simulink model "model_r2016b"  (R2016b)
settings: Solver=VariableStepAuto  StartTime=0.0  StopTime=10.0  RelTol=1e-6
values from neighbouring files (symbols this model uses):
  a = 1.1    [Youla_controller.mat]    (also in parameters.m)
  b = 1.68    [Youla_controller.mat]    (also in parameters.m)
  b_hsf = 22.9183118052    [Youla_controller.mat]    (also in extendedKalmanFilter.m = obj.b_hsf; parameters.m; unscentedKalmanFilter.m = obj.b_hsf)
  b_hsf_RL = 45.8366236105    [Youla_controller.mat]    (also in parameters.m)
  b_hsf_RR = 45.8366236105    [Youla_controller.mat]    (also in parameters.m)
  b_sf_R = 45.8366236105    [Youla_controller.mat]    (also in parameters.m)
  chassis_state_init = [U_0 0 0 U_0/rw U_0/rw U_0/rw U_0/rw 0 0 0]    [main.m]
  Cx = 43302.5    [Youla_controller.mat]    (also in parameters.m; sandbox.m = CRx)
  Cy = 28427.8739632    [Youla_controller.mat]    (also in parameters.m; sandbox.m = CRy)
  DFFy = 310.189835229    [Youla_controller.mat]    (also in parameters.m)
  DFRy = 203.100487352    [Youla_controller.mat]    (also in parameters.m)
  DFx = 143.09352518    [Youla_controller.mat]    (also in parameters.m)
  fFLz0 = 4535.18417266    [Youla_controller.mat]    (also in parameters.m)
  fFRz0 = 4535.18417266    [Youla_controller.mat]    (also in parameters.m)
  fRLz0 = 2969.46582734    [Youla_controller.mat]    (also in extendedKalmanFilter.m = obj.fRLz0; parameters.m; unscentedKalmanFilter.m = obj.fRLz0)
  fRRz0 = 2969.46582734    [Youla_controller.mat]    (also in extendedKalmanFilter.m = obj.fRRz0; parameters.m; unscentedKalmanFilter.m = obj.fRRz0)
  G = minreal(C*inv(s*eye(4)-A)*B + D,1e-9)    [Youla_design.m]    (also in extendedKalmanFilter.m = obj.G; parameters.m = 9.96488294314; unscentedKalmanFilter.m = obj.G)
  J_hsf = 0.009    [Youla_controller.mat]    (also in parameters.m)
  Jm_R = 0.0351    [Youla_controller.mat]    (also in extendedKalmanFilter.m = obj.Jm_R; parameters.m; unscentedKalmanFilter.m = obj.Jm_R)
  Jw = 0.9    [Youla_controller.mat]    (also in extendedKalmanFilter.m = obj.Jw; parameters.m; unscentedKalmanFilter.m = obj.Jw)
  Jy = 2315.3    [Youla_controller.mat]    (also in parameters.m)
  K_hsf = 2291.83118052    [Youla_controller.mat]    (also in extendedKalmanFilter.m = obj.K_hsf; parameters.m; unscentedKalmanFilter.m = obj.K_hsf)
  K_hsf_RL = 4583.66236105    [Youla_controller.mat]    (also in parameters.m)
  K_hsf_RR = 4583.66236105    [Youla_controller.mat]    (also in parameters.m)
  K_sf_R = 11459.1559026    [Youla_controller.mat]    (also in parameters.m)
  m = 1530    [Youla_controller.mat]    (also in extendedKalmanFilter.m = obj.m; parameters.m; unscentedKalmanFilter.m = obj.m)
  rear_axle_state_init = [G*U_0/rw 0]    [main.m]
  rw = 0.325    [Youla_controller.mat]    (also in extendedKalmanFilter.m = obj.rw; parameters.m; unscentedKalmanFilter.m = obj.rw)
  T = 1.55    [Youla_controller.mat]    (also in parameters.m; sandbox.m = 1.42857142857)
  U_0 = 100/3.6    (= 27.7777777778)    [main.m]
libraries: cstblocks x1
settings Model: Creator=louis  LastModifiedBy=louis

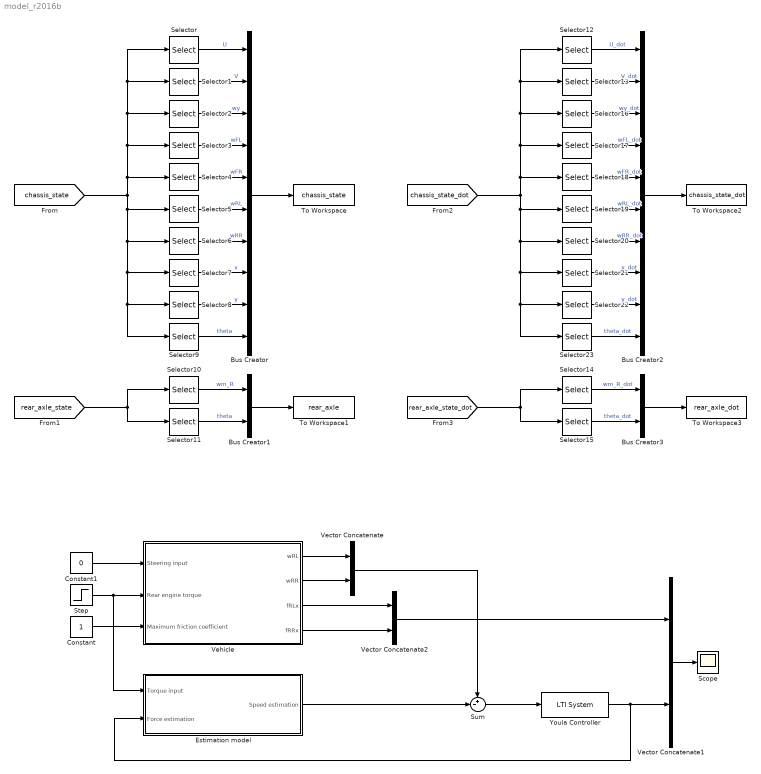
== system model_r2016b ==
  Bus Creator : BusCreator  Inputs=10
  Bus Creator1 : BusCreator  Inputs=2
  Bus Creator2 : BusCreator  Inputs=10
  Bus Creator3 : BusCreator  Inputs=2
  Constant : Constant
  Constant1 : Constant  Value=0
  Estimation model : Subsystem
  Scope : Scope
  Selector{,10,12,14} (4 alike) : Selector  IndexOptions=Index vector (dialog)  Indices=1  OutputSizes=1
  Selector{1,11,13,15} (4 alike) : Selector  IndexOptions=Index vector (dialog)  Indices=2  OutputSizes=1
  Selector16 : Selector  IndexOptions=Index vector (dialog)  Indices=3  OutputSizes=1
  Selector17 : Selector  IndexOptions=Index vector (dialog)  Indices=4  OutputSizes=1
  Selector18 : Selector  IndexOptions=Index vector (dialog)  Indices=5  OutputSizes=1
  Selector19 : Selector  IndexOptions=Index vector (dialog)  Indices=6  OutputSizes=1
  Selector2 : Selector  IndexOptions=Index vector (dialog)  Indices=3  OutputSizes=1
  Selector20 : Selector  IndexOptions=Index vector (dialog)  Indices=7  OutputSizes=1
  Selector21 : Selector  IndexOptions=Index vector (dialog)  Indices=8  OutputSizes=1
  Selector22 : Selector  IndexOptions=Index vector (dialog)  Indices=9  OutputSizes=1
  Selector23 : Selector  IndexOptions=Index vector (dialog)  Indices=10  OutputSizes=1
  Selector3 : Selector  IndexOptions=Index vector (dialog)  Indices=4  OutputSizes=1
  Selector4 : Selector  IndexOptions=Index vector (dialog)  Indices=5  OutputSizes=1
  Selector5 : Selector  IndexOptions=Index vector (dialog)  Indices=6  OutputSizes=1
  Selector6 : Selector  IndexOptions=Index vector (dialog)  Indices=7  OutputSizes=1
  Selector7 : Selector  IndexOptions=Index vector (dialog)  Indices=8  OutputSizes=1
  Selector8 : Selector  IndexOptions=Index vector (dialog)  Indices=9  OutputSizes=1
  Selector9 : Selector  IndexOptions=Index vector (dialog)  Indices=10  OutputSizes=1
  Step : Step  After=50  SampleTime=0
  Sum : Sum  Inputs=+-|
  To Workspace : ToWorkspace  VariableName=chassis_state  SaveFormat=Timeseries  SampleTime=-1
  To Workspace1 : ToWorkspace  VariableName=rear_axle  SaveFormat=Timeseries  SampleTime=-1
  To Workspace2 : ToWorkspace  VariableName=chassis_state_dot  SaveFormat=Timeseries  SampleTime=-1
  To Workspace3 : ToWorkspace  VariableName=rear_axle_dot  SaveFormat=Timeseries  SampleTime=-1
  Vector Concatenate : Concatenate
  Vector Concatenate1 : Concatenate
  Vector Concatenate2 : Concatenate
  Vehicle : Subsystem
  Youla Controller : cstblocks/LTI System  sys=Gc  IC=[]
  wires:
  [chassis_state] -> Selector4/1, Selector3/1, Selector2/1, Selector1/1, Selector/1, Selector5/1, Selector6/1, Selector7/1, Selector8/1, Selector9/1
  Selector/1 -> Bus Creator/1  "U"
  Selector9/1 -> Bus Creator/10  "theta"
  Selector8/1 -> Bus Creator/9  "y"
  Selector7/1 -> Bus Creator/8  "x"
  Selector6/1 -> Bus Creator/7  "wRR"
  Selector5/1 -> Bus Creator/6  "wRL"
  Bus Creator/1 -> To Workspace/1
  Selector1/1 -> Bus Creator/2  "V"
  Selector2/1 -> Bus Creator/3  "wy"
  Selector3/1 -> Bus Creator/4  "wFL"
  Selector4/1 -> Bus Creator/5  "wFR"
  Selector11/1 -> Bus Creator1/2  "theta"
  Bus Creator1/1 -> To Workspace1/1
  [rear_axle_state] -> Selector11/1, Selector10/1
  Selector10/1 -> Bus Creator1/1  "wm_R"
  Selector12/1 -> Bus Creator2/1  "U_dot"
  [chassis_state_dot] -> Selector18/1, Selector17/1, Selector16/1, Selector13/1, Selector12/1, Selector19/1, Selector20/1, Selector21/1, Selector22/1, Selector23/1
  Selector22/1 -> Bus Creator2/9  "y_dot"
  Selector20/1 -> Bus Creator2/7  "wRR_dot"
  Selector18/1 -> Bus Creator2/5  "wFR_dot"
  Bus Creator2/1 -> To Workspace2/1
  Selector16/1 -> Bus Creator2/3  "wy_dot"
  Bus Creator3/1 -> To Workspace3/1
  Selector13/1 -> Bus Creator2/2  "V_dot"
  Selector21/1 -> Bus Creator2/8  "x_dot"
  Selector23/1 -> Bus Creator2/10  "theta_dot"
  Selector19/1 -> Bus Creator2/6  "wRL_dot"
  [rear_axle_state_dot] -> Selector15/1, Selector14/1
  Selector15/1 -> Bus Creator3/2  "theta_dot"
  Selector17/1 -> Bus Creator2/4  "wFL_dot"
  Selector14/1 -> Bus Creator3/1  "wm_R_dot"
  Constant/1 -> Vehicle/3(Maximum friction coefficient)
  Constant1/1 -> Vehicle/1(Steering input)
  Step/1 -> Estimation model/1(Torque input), Vehicle/2(Rear engine torque)
  Vehicle/1(wRL) -> Vector Concatenate/1
  Vehicle/2(wRR) -> Vector Concatenate/2
  Sum/1 -> Youla Controller/1
  Vector Concatenate/1 -> Sum/1
  Youla Controller/1 -> Estimation model/2(Force estimation), Vector Concatenate1/2
  Estimation model/1(Speed estimation) -> Sum/2
  Vector Concatenate1/1 -> Scope/1
  Vehicle/3(fRLx) -> Vector Concatenate2/1
  Vehicle/4(fRRx) -> Vector Concatenate2/2
  Vector Concatenate2/1 -> Vector Concatenate1/1

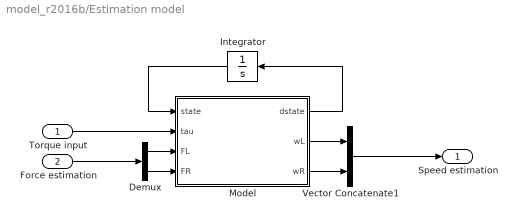
== system model_r2016b/Estimation model ==
  Torque input : Inport
  Force estimation : Inport  Port=2
  Demux : Demux  Outputs=2
  Integrator : Integrator  InitialCondition=[U_0/rw*G 0 U_0/rw U_0/rw]
  Model : MATLAB Function  TreatAsAtomicUnit=on
  Vector Concatenate1 : Concatenate
  Speed estimation : Outport
  wires:
  Demux/1 -> Model/3(FL)
  Vector Concatenate1/1 -> Speed estimation/1
  Integrator/1 -> Model/1(state)
  Model/3(wR) -> Vector Concatenate1/2
  Force estimation/1 -> Demux/1
  Model/2(wL) -> Vector Concatenate1/1
  Demux/2 -> Model/4(FR)
  Torque input/1 -> Model/2(tau)
  Model/1(dstate) -> Integrator/1

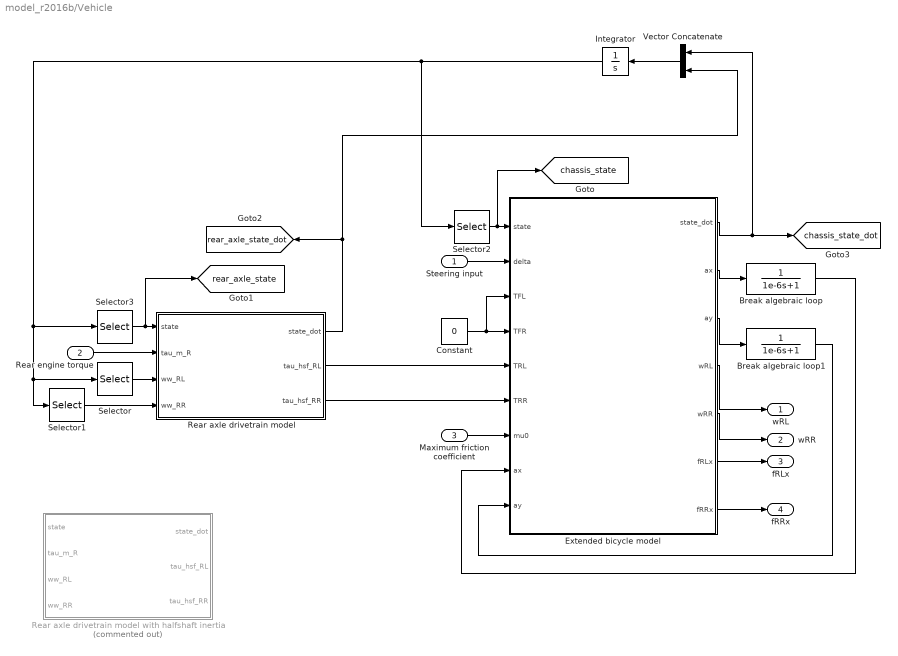
== system model_r2016b/Vehicle ==
  Steering input : Inport
  Rear engine torque : Inport  Port=2
  Maximum friction coefficient : Inport  Port=3
  Break algebraic loop : TransferFcn  Denominator=[1e-6 1]
  Break algebraic loop1 : TransferFcn  Denominator=[1e-6 1]
  Constant : Constant  Value=0
  Extended bicycle model : MATLAB Function  TreatAsAtomicUnit=on
  Integrator : Integrator  InitialCondition=[chassis_state_init rear_axle_state_init]
  Rear axle drivetrain model : MATLAB Function  TreatAsAtomicUnit=on
  Rear axle drivetrain model with halfshaft inertia : MATLAB Function  Commented=on  TreatAsAtomicUnit=on
  Selector : Selector  IndexOptions=Index vector (dialog)  Indices=[6]  OutputSizes=1
  Selector1 : Selector  IndexOptions=Index vector (dialog)  Indices=[7]  OutputSizes=1
  Selector2 : Selector  IndexOptions=Index vector (dialog)  Indices=[1:10]  OutputSizes=1
  Selector3 : Selector  IndexOptions=Index vector (dialog)  Indices=[11:12]  OutputSizes=1
  Vector Concatenate : Concatenate
  wRL : Outport
  wRR : Outport  Port=2
  fRLx : Outport  Port=3
  fRRx : Outport  Port=4
  tag scope: chassis_state=global, chassis_state_dot=global, rear_axle_state=global, rear_axle_state_dot=global
  wires:
  Maximum friction coefficient/1 -> Extended bicycle model/7(mu0)
  Steering input/1 -> Extended bicycle model/2(delta)
  Rear engine torque/1 -> Rear axle drivetrain model/2(tau_m_R)
  Extended bicycle model/3(ay) -> Break algebraic loop1/1
  Integrator/1 -> Selector2/1, Selector3/1, Selector1/1, Selector/1
  Rear axle drivetrain model/2(tau_hsf_RL) -> Extended bicycle model/5(TRL)
  Extended bicycle model/1(state_dot) -> Vector Concatenate/1, [chassis_state_dot]
  Rear axle drivetrain model/3(tau_hsf_RR) -> Extended bicycle model/6(TRR)
  Break algebraic loop1/1 -> Extended bicycle model/9("ay ")
  Break algebraic loop/1 -> Extended bicycle model/8("ax ")
  Extended bicycle model/2(ax) -> Break algebraic loop/1
  Constant/1 -> Extended bicycle model/4(TFR), Extended bicycle model/3(TFL)
  Selector1/1 -> Rear axle drivetrain model/4(ww_RR)
  Selector/1 -> Rear axle drivetrain model/3(ww_RL)
  Rear axle drivetrain model/1(state_dot) -> [rear_axle_state_dot], Vector Concatenate/2
  Vector Concatenate/1 -> Integrator/1
  Selector2/1 -> [chassis_state], Extended bicycle model/1(state)
  Selector3/1 -> [rear_axle_state], Rear axle drivetrain model/1(state)
  Extended bicycle model/4(wRL) -> wRL/1
  Extended bicycle model/5(wRR) -> wRR/1
  Extended bicycle model/6(fRLx) -> fRLx/1
  Extended bicycle model/7(fRRx) -> fRRx/1

== matlab function model_r2016b/Vehicle/Rear axle drivetrain model with halfshaft inertia ==
  data: state input; state_dot output; tau_m_R input; ww_RL input; ww_RR input; tau_hsf_RL output; tau_hsf_RR output; Jm_R parameter; J_hsf parameter; K_sf_R parameter; b_sf_R parameter; K_hsf_RL parameter; b_hsf_RL parameter; K_hsf_RR parameter; b_hsf_RR parameter; G parameter
function [state_dot, tau_hsf_RL, tau_hsf_RR] = ... 
    rearAxleModel(state, tau_m_R, ww_RL, ww_RR,...
    Jm_R, J_hsf, K_sf_R, b_sf_R, ...
    K_hsf_RL, b_hsf_RL, K_hsf_RR, b_hsf_RR, G) ...

%% Rename the states
wm_R         = state(1);    % Angular velocity of the rear shaft 
wh_RL        = state(2);    % Rear left halfshaft angular velocity
wh_RR        = state(3);    % Rear right halfshaft angular velocity
theta_hsf_RL = state(4);    % Rear left  axle halfshaft displacement 
theta_hsf_RR = state(5);    % Rear right axle halfshaft displacement
theta_sf_R   = state(6);    % Rear motor axle halfshaft displacement 

%% Shaft torque
tau_hsf_RL = K_hsf_RL * theta_hsf_RL + b_hsf_RL * (wh_RL - ww_RL); 
tau_hsf_RR = K_hsf_RR * theta_hsf_RR + b_hsf_RR * (wh_RR - ww_RR);
tau_sf_R   = K_sf_R   * theta_sf_R   + b_sf_R   * (wm_R - G/2*(wh_RL + wh_RR));

%% Compute the time derivatives
wm_rear_dot = 1/Jm_R * (tau_m_R - tau_sf_R);  
wh_RL_dot   = 1/J_hsf * (G*tau_sf_R/2 - tau_hsf_RL);
wh_RR_dot   = 1/J_hsf * (G*tau_sf_R/2 - tau_hsf_RR);
theta_hsf_RL_dot = wh_RL - ww_RL;
theta_hsf_RR_dot = wh_RR - ww_RR;
theta_sf_R_dot   = wm_R - G/2 * (wh_RL + wh_RR);

%% Return the state time derivative 
state_dot = [wm_rear_dot; wh_RL_dot; wh_RR_dot; theta_hsf_RL_dot;
    theta_hsf_RR_dot; theta_sf_R_dot];

end

== matlab function model_r2016b/Vehicle/Extended bicycle model ==
  data: state input; delta input; TFL input; TFR input; TRL input; TRR input; mu0 input; state_dot output; ax input; ay input; ax output; ay output; m parameter; Jy parameter; Jw parameter; a parameter; b parameter; T parameter; rw parameter; Cx parameter; Cy parameter; eps parameter; fFLz0 parameter; fFRz0 parameter; fRLz0 parameter; fRRz0 parameter; DFx parameter; DFFy parameter; DFRy parameter; wRL output; wRR output; fRLx output; fRRx output
function [state_dot,ax,ay,wRL,wRR,fRLx,fRRx] = vehicleEOM(state,delta,TFL,TFR,TRL,TRR,mu0,ax,ay,m,Jy,...
    Jw,a,b,T,rw,Cx,Cy,eps,fFLz0,fFRz0,fRLz0,fRRz0,DFx,DFFy,DFRy)

%% Rename the states
U     = state(1);
V     = state(2);
wy    = state(3);
wFL   = state(4);
wFR   = state(5);
wRL   = state(6);
wRR   = state(7);
theta = state(10);

%% Compute tire forces
% Wheel velocities
vFLxc = U - T*wy/2;
vFLyc = V + a*wy;
vFRxc = U + T*wy/2;
vFRyc = V + a*wy;
% Rotate to obtain velocities in the tire frame
vFLx =  vFLxc * cos(delta) + vFLyc * sin(delta);
vFLy = -vFLxc * sin(delta) + vFLyc * cos(delta);
vFRx =  vFRxc * cos(delta) + vFRyc * sin(delta);
vFRy = -vFRxc * sin(delta) + vFRyc * cos(delta);

vRLx = U - T*wy/2;
vRLy = V - b*wy;
vRRx = U + T*wy/2;
vRRy = V - b*wy;

% Wheel slip
% FL wheel
if abs(rw*wFL) > abs(vFLx)
    den = rw*wFL;
else
    den = vFLx;
end
if den == 0
    sFLx = 0;
else
    sFLx = -(vFLx - rw * wFL) / den;
end
% FR wheel
if abs(rw*wFR) > abs(vFRx)
    den = rw*wFR;
else
    den = vFRx;
end
if den == 0
    sFRx = 0;
else
    sFRx = -(vFRx - rw * wFR) / den;
end

% RL wheel
if abs(rw*wRL) > abs(vRLx)
    den = rw*wRL;
else
    den = vRLx;
end
if den == 0
    sRLx = 0;
else
    sRLx = -(vRLx - rw * wRL) / den;
end

% RR wheel
if abs(rw*wRR) > abs(vRRx)
    den = rw*wRR;
else
    den = vRRx;
end
if den == 0
    sRRx = 0;
else
    sRRx = -(vRRx - rw * wRR) / den;
end

% Slip angle
% FL wheel
if vFLx == 0
    if vFLy == 0
        alphaFL = 0;
    else
        alphaFL = -sign(vFLy)*pi/2;
    end
else
    alphaFL = - atan(vFLy/abs(vFLx));
end

% FR wheel
if vFRx == 0
    if vFRy == 0
        alphaFR = 0;
    else
        alphaFR = -sign(vFRy)*pi/2;
    end
else
    alphaFR = - atan(vFRy/abs(vFRx));
end

% RL wheel
if vRLx == 0
    if vRLy == 0
        alphaRL = 0;
    else
        alphaRL = -sign(vRLy)*pi/2;
    end
else
    alphaRL = - atan(vRLy/abs(vRLx));
end

% RR wheel
if vRRx == 0
    if vRRy == 0
        alphaRR = 0;
    else
        alphaRR = -sign(vRRy)*pi/2;
    end
else
    alphaRR = - atan(vRRy/abs(vRRx));
end

% Normal forces
fFLz = fFLz0 - DFx*ax - DFFy*ay;
fFRz = fFRz0 - DFx*ax + DFFy*ay;
fRLz = fRLz0 + DFx*ax - DFRy*ay;
fRRz = fRRz0 + DFx*ax + DFRy*ay;

% % Static normal force (for debugging)
% fFLz = fFLz0;
% fFRz = fFRz0;
% fRLz = fRLz0;
% fRRz = fRRz0;

% Tire forces
[fFLxt,fFLyt] = Dugoff(Cx,Cy,fFLz,sFLx,alphaFL,vFLx,mu0,eps);
[fFRxt,fFRyt] = Dugoff(Cx,Cy,fFRz,sFRx,alphaFR,vFRx,mu0,eps);
[fRLx,fRLy]   = Dugoff(Cx,Cy,fRLz,sRLx,alphaRL,vRLx,mu0,eps);
[fRRx,fRRy]   = Dugoff(Cx,Cy,fRRz,sRRx,alphaRR,vRRx,mu0,eps);

% % Linear tire model (for debugging)
% fFLxt = Cx * sFLx;
% fFRxt = Cx * sFRx;
% fRLx  = Cx * sRLx;
% fRRx  = Cx * sRRx;
% fFLyt = Cy * alphaFL;
% fFRyt = Cy * alphaFR;
% fRLy  = Cy * alphaRL;
% fRRy  = Cy * alphaRR;

% Rotate to obtain forcces in the chassis frame
fFLx = fFLxt * cos(delta) - fFLyt * sin(delta);
fFLy = fFLxt * sin(delta) + fFLyt * cos(delta);
fFRx = fFRxt * cos(delta) - fFRyt * sin(delta);
fFRy = fFRxt * sin(delta) + fFRyt * cos(delta);


%% Compute the time derivatives
U_dot     = 1/m * (fFLx + fFRx + fRLx + fRRx + m*V*wy);
V_dot     = 1/m * (fFLy + fFRy + fRLy + fRRy - m*U*wy);
wy_dot    = 1/Jy * (a * (fFLy + fFRy) - b * (fRLy + fRRy)...
    + T/2 * (fFRx - fFLx + fRRx - fRLx));
x_dot     = U * cos(theta) - V * sin(theta);
y_dot     = U * sin(theta) + V * cos(theta);
theta_dot = wy;

wFL_dot = (TFL - rw * fFLxt)/Jw;
wFR_dot = (TFR - rw * fFRxt)/Jw;
wRL_dot = (TRL - rw * fRLx) /Jw;
wRR_dot = (TRR - rw * fRRx) /Jw;

%% Return the state time derivative
state_dot = [U_dot;V_dot;wy_dot;wFL_dot;wFR_dot;wRL_dot;wRR_dot;
    x_dot;y_dot;theta_dot];

%% Update acceleration
ax = U_dot - V*wy;
ay = V_dot + U*wy;

%% Return other variables

end

== matlab function model_r2016b/Estimation model/Model ==
  data: state input; dstate output; tau input; FL input; FR input; K_hsf parameter; b_hsf parameter; G parameter; rw parameter; Jm_R parameter; wL output; wR output
function [dstate,wL,wR] = estimationModel(state,tau,FL,FR,K_hsf, b_hsf, G, rw, Jm_R)

wm      = state(1);
the_hsr = state(2);
wL      = state(3);
wR      = state(4);

tau_hsr = K_hsf*the_hsr + b_hsf*(2/G * wm - wL - wR);

dwm = (tau-2*tau_hsr/G)/Jm_R;
dthe_hsr = 2*wm/G - wL - wR;
dwL = (tau_hsr-rw*FL);
dwR = (tau_hsr-rw*FR);

dstate = [dwm, dthe_hsr, dwL, dwR];

== matlab function model_r2016b/Vehicle/Rear axle drivetrain model ==
  data: state input; state_dot output; tau_m_R input; ww_RL input; ww_RR input; tau_hsf_RL output; tau_hsf_RR output; Jm_R parameter; K_hsf parameter; b_hsf parameter; G parameter
function [state_dot, tau_hsf_RL, tau_hsf_RR] = ... 
    rearAxleModel(state, tau_m_R, ww_RL, ww_RR,...
    Jm_R, K_hsf, b_hsf, G) ...

%% Rename the states
wm_R      = state(1);   % Angular velocity of the rear shaft 
theta_hsf = state(2);   % Halfshaft displacement 

%% Shaft torque
tau_hsf = K_hsf * theta_hsf + b_hsf * (2/G*wm_R - ww_RL - ww_RR); 

%% Compute the time derivatives
wm_R_dot      = 1/Jm_R * (tau_m_R - 2/G * tau_hsf);  
theta_hsf_dot = 2/G * wm_R - ww_RL - ww_RR;

%% Return the state time derivative 
state_dot = [wm_R_dot; theta_hsf_dot];

%% Return the halfshaft torque
tau_hsf_RL = tau_hsf;
tau_hsf_RR = tau_hsf;

end
